simulink model "poleVaultSim"  (R2024a)
settings: Solver=VariableStepAuto  StartTime=0.0  StopTime=4  MaxStep=.0002  RelTol=1e-3  EnableMultiTasking=on
undefined symbols (not defined in the file or in its folder): k, theta0
libraries: simulink_extras x4
settings Model: PauseTimes=1.31  PacingRate=0.500000  Creator=amitraj  LastModifiedBy=grouleau
settings SolverCC: AlgebraicLoopSolver=TrustRegion
settings OptimizationCC: LifeSpan=inf
settings DebuggingCC: UnconnectedInputMsg=warning  UnconnectedOutputMsg=warning  UnconnectedLineMsg=warning  SFUnexpectedBacktrackingDiag=warning  SFNoUnconditionalDefaultTransitionDiag=warning  ArithmeticOperatorsInVariantConditions=warning
settings ModelReferenceCC: EnableRefExpFcnMdlSchedulingChecks=on
settings SFSimCC: SimUseLocalCustomCode=off  CustomCodeUndefinedFunction=UseInterfaceOnly
settings RTWCC: RTWUseLocalCustomCode=off  GPUComputeCapability=3.5
settings CodeAppCC: StateflowObjectComments=on
settings GRTTargetCC: TargetLangStandard=C89/C90 (ANSI)
settings ConfigComp: CovMetricSettings=dw  CovSaveCumulativeToWorkspaceVar=on  CovSaveSingleToWorkspaceVar=on  CovExternalEMLEnable=off

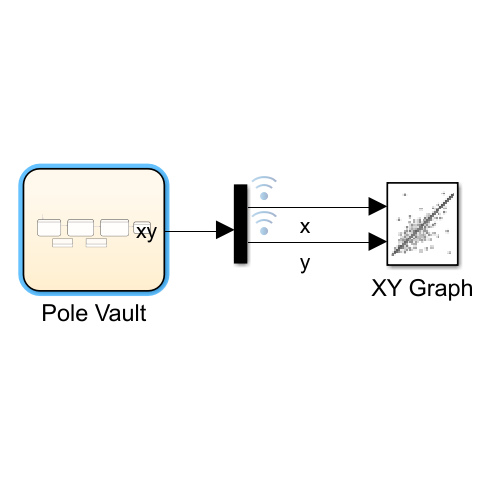
[thumbnail: Simulink's stored preview of the top-level diagram]
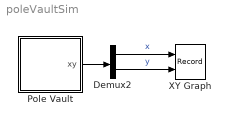
== system poleVaultSim ==
  Demux2 : Demux  Outputs=2
  Pole Vault : Stateflow chart  TreatAsAtomicUnit=on
  XY Graph : Record  FileSettingsInternal="{\"entries\":[{\"content\":{\"excelSettings\":{\"content\":{},\"type\":\"Streamout.ExcelSettings\"}},\"type\":\"Streamout.FileSettingStorage\",\"uuid\":\"\"}],\"packageUris\":[\"http:\\/\\/schema.mathworks.com\\/mf0\\/streamout_blocks\\/R2020a\"],\"version\":\"1.0\"}"  Layout=[1 1]  SignalsInternal="{\"entries\":[{\"content\":{\"signals\":[{\"content\":{\"blockPath\":[],\"dimensions\":[1],\"domain\":\"\",\"lineColor\":\"#a2142f\",\"plots\":[ 1 ],\"port\":1,\"sid\":[\"\"],\"signalID\":1,\"signalName\":\"x\"},\"type\":\"RecordBlkView.Signal\",\"uuid\":\"\"},{\"content\":{\"blockPath\":[],\"dimensions\":[1],\"domain\":\"\",\"lineColor\":\"#139fff\",\"plots\":[ 1 ],\"port\":2,\"sid\":[\"\"],\"signalID\":2,\"signalName\":\"y\"},\"type\":\"RecordBlkView.Signal\",\"uuid\":\"\"}]},\"type\":\"RecordBlkView.InputSignals\",\"uuid\":\"\"}],\"packageUris\":[\"http:\\/\\/schema.mathworks.com\\/mf0\\/streamout_blocks\\/R2020a\"],\"version\":\"1.0\"}"  VisualizationBindings="{\"xyplotplugin\":{\"info\":[{\"series\":[{\"bindingParametersList\":[{\"parameter\":\"X-Axis\",\"signalID\":1,\"signalName\":\"x\"},{\"parameter\":\"Y-Axis\",\"signalID\":2,\"signalName\":\"y\"}],\"seriesID\":0}],\"subplotID\":1}]}}"  CompatibilityTag=XY  st=-1
  wires:
  Demux2/1 -> XY Graph/1  "x"
  Demux2/2 -> XY Graph/2  "y"
  Pole Vault/1(xy) -> Demux2/1

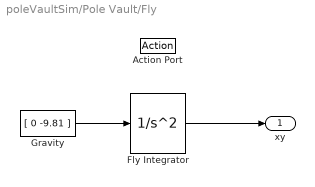
== system poleVaultSim/Pole Vault/Fly ==
  Action Port : ActionPort
      settings: CopyFcn=Stateflow.SLINSF.SimulinkMan.removeBlockPreDeleteFcn  PreDeleteFcn=Stateflow.SLINSF.SimulinkMan.unsafePredeleteFcn
  Fly Integrator : SecondOrderIntegrator  StateNameX='x'  StateNameDXDT='dx'  ShowOutput=x
  Gravity : Constant  Value=[ 0 -9.81 ]
  xy : Outport
  wires:
  Gravity/1 -> Fly Integrator/1
  Fly Integrator/1 -> xy/1

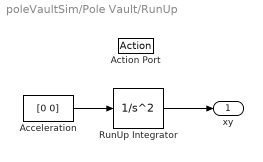
== system poleVaultSim/Pole Vault/RunUp ==
  Action Port : ActionPort
      settings: CopyFcn=Stateflow.SLINSF.SimulinkMan.removeBlockPreDeleteFcn  PreDeleteFcn=Stateflow.SLINSF.SimulinkMan.unsafePredeleteFcn
  Acceleration : Constant  Value=[0 0]
  RunUp Integrator : SecondOrderIntegrator  ICX=[10 1]  StateNameX='x'  ICDXDT=[-10 0]  StateNameDXDT='dx'  ShowOutput=x
      settings: AttributesFormatString=|
      | Initial Position: %<ICX>
      | Initial Velocity%<ICDXDT>
  xy : Outport
  wires:
  Acceleration/1 -> RunUp Integrator/1
  RunUp Integrator/1 -> xy/1

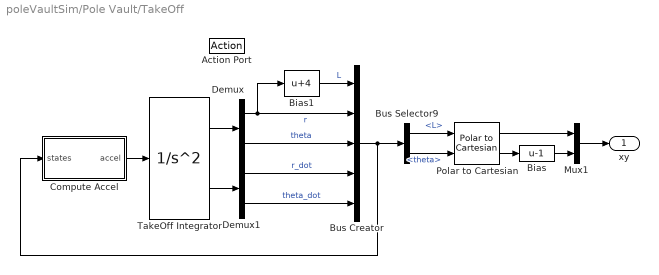
== system poleVaultSim/Pole Vault/TakeOff ==
  Action Port : ActionPort
      settings: CopyFcn=Stateflow.SLINSF.SimulinkMan.removeBlockPreDeleteFcn  PreDeleteFcn=Stateflow.SLINSF.SimulinkMan.unsafePredeleteFcn
  Bias : Bias  Bias=-1  SaturateOnIntegerOverflow=off
  Bias1 : Bias  Bias=4  SaturateOnIntegerOverflow=off
  Bus Creator : BusCreator  Inputs=5
  Bus Selector9 : BusSelector  OutputSignals=L,theta
  Compute Accel : Subsystem
  Demux : Demux  Outputs=2
  Demux1 : Demux  Outputs=2
  Mux1 : Mux  Inputs=2
  Polar to Cartesian : simulink_extras/Transformations/Polar to Cartesian
  TakeOff Integrator : SecondOrderIntegrator  StateNameX='x'  StateNameDXDT='dx'
  xy : Outport
  wires:
  Compute Accel/1(accel) -> TakeOff Integrator/1
  Bias/1 -> Mux1/2
  Demux1/1 -> Bus Creator/4  "r_dot"
  Polar to Cartesian/2 -> Bias/1
  Bus Selector9/1 -> Polar to Cartesian/1  "<L>"
  Mux1/1 -> xy/1
  Bus Selector9/2 -> Polar to Cartesian/2  "<theta>"
  TakeOff Integrator/1 -> Demux/1
  Polar to Cartesian/1 -> Mux1/1
  Bias1/1 -> Bus Creator/1  "L"
  Demux1/2 -> Bus Creator/5  "theta_dot"
  Bus Creator/1 -> Compute Accel/1(states), Bus Selector9/1
  Demux/1 -> Bus Creator/2, Bias1/1  "r"
  Demux/2 -> Bus Creator/3  "theta"
  TakeOff Integrator/2 -> Demux1/1

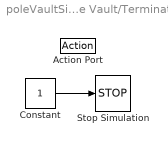
== system poleVaultSim/Pole Vault/Terminate ==
  Action Port : ActionPort
      settings: CopyFcn=Stateflow.SLINSF.SimulinkMan.removeBlockPreDeleteFcn  PreDeleteFcn=Stateflow.SLINSF.SimulinkMan.unsafePredeleteFcn
  Constant : Constant
  Stop Simulation : Stop
  wires:
  Constant/1 -> Stop Simulation/1

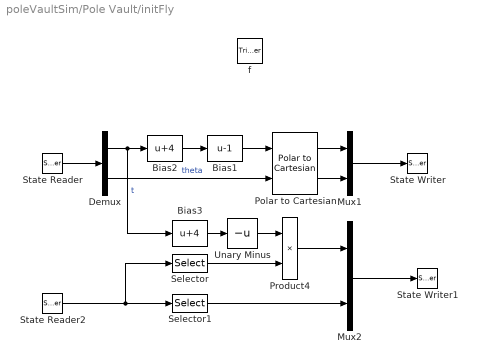
== system poleVaultSim/Pole Vault/initFly ==
  f : TriggerPort  TriggerType=function-call  VariantControl=(inherit)
      settings: CopyFcn=Stateflow.SLINSF.SimulinkMan.removeBlockPreDeleteFcn  PreDeleteFcn=Stateflow.SLINSF.SimulinkMan.unsafePredeleteFcn
  Bias1 : Bias  Bias=-1  SaturateOnIntegerOverflow=off
  Bias2 : Bias  Bias=4  SaturateOnIntegerOverflow=off
  Bias3 : Bias  Bias=4  SaturateOnIntegerOverflow=off
  Demux : Demux  Outputs=2
  Mux1 : Mux  Inputs=2
  Mux2 : Mux  Inputs=2
  Polar to Cartesian : simulink_extras/Transformations/Polar to Cartesian
  Product4 : Product
  Selector : Selector  InputPortWidth=2  IndexOptions=Index vector (dialog)  Indices=2  OutputSizes=1
  Selector1 : Selector  InputPortWidth=2  IndexOptions=Index vector (dialog)  Indices=1  OutputSizes=1
  State Reader : StateReader  StateOwnerBlock=../../TakeOff/TakeOff Integrator  StateName=x
  State Reader2 : StateReader  StateOwnerBlock=../../TakeOff/TakeOff Integrator  StateName=dx
  State Writer : StateWriter  StateOwnerBlock=../../Fly/Fly Integrator  StateName=x
  State Writer1 : StateWriter  StateOwnerBlock=../../Fly/Fly Integrator  StateName=dx
  Unary Minus : UnaryMinus
  wires:
  Bias2/1 -> Bias1/1
  Polar to Cartesian/1 -> Mux1/1
  Mux1/1 -> State Writer/1
  Bias1/1 -> Polar to Cartesian/1
  Polar to Cartesian/2 -> Mux1/2
  Demux/2 -> Polar to Cartesian/2  "theta"
  Product4/1 -> Mux2/1
  Selector1/1 -> Mux2/2
  Bias3/1 -> Unary Minus/1
  Mux2/1 -> State Writer1/1
  Unary Minus/1 -> Product4/1
  Demux/1 -> Bias3/1, Bias2/1  "t"
  State Reader/1 -> Demux/1
  Selector/1 -> Product4/2
  State Reader2/1 -> Selector/1, Selector1/1

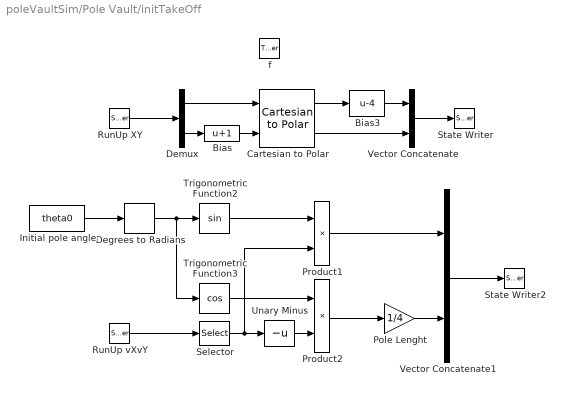
== system poleVaultSim/Pole Vault/initTakeOff ==
  f : TriggerPort  TriggerType=function-call  VariantControl=(inherit)
      settings: CopyFcn=Stateflow.SLINSF.SimulinkMan.removeBlockPreDeleteFcn  PreDeleteFcn=Stateflow.SLINSF.SimulinkMan.unsafePredeleteFcn
  Bias : Bias  Bias=1  SaturateOnIntegerOverflow=off
  Bias3 : Bias  Bias=-4  SaturateOnIntegerOverflow=off
  Cartesian to Polar : simulink_extras/Transformations/Cartesian to Polar
  Degrees to Radians : simulink_extras/Transformations/Degrees to Radians
  Demux : Demux  Outputs=2
  Initial pole angle : Constant  Value=theta0
  Pole Lenght : Gain  Gain=1/4
  Product1 : Product
  Product2 : Product
  RunUp XY : StateReader  StateOwnerBlock=../../RunUp/RunUp Integrator  StateName=x
  RunUp vXvY : StateReader  StateOwnerBlock=../../RunUp/RunUp Integrator  StateName=dx
  Selector : Selector  InputPortWidth=2  IndexOptions=Index vector (dialog)  Indices=1  OutputSizes=1
  State Writer : StateWriter  StateOwnerBlock=../../TakeOff/TakeOff Integrator  StateName=x
  State Writer2 : StateWriter  StateOwnerBlock=../../TakeOff/TakeOff Integrator  StateName=dx
  Trigonometric Function2 : Trigonometry
  Trigonometric Function3 : Trigonometry  Operator=cos
  Unary Minus : UnaryMinus
  Vector Concatenate : Concatenate
  Vector Concatenate1 : Concatenate
  wires:
  Unary Minus/1 -> Product2/2
  Product2/1 -> Pole Lenght/1
  RunUp vXvY/1 -> Selector/1
  Trigonometric Function3/1 -> Product2/1
  Trigonometric Function2/1 -> Product1/1
  Cartesian to Polar/1 -> Bias3/1
  Initial pole angle/1 -> Degrees to Radians/1
  Demux/1 -> Cartesian to Polar/1
  Demux/2 -> Bias/1
  Selector/1 -> Product1/2, Unary Minus/1
  Bias/1 -> Cartesian to Polar/2
  Pole Lenght/1 -> Vector Concatenate1/2
  RunUp XY/1 -> Demux/1
  Bias3/1 -> Vector Concatenate/1
  Cartesian to Polar/2 -> Vector Concatenate/2
  Vector Concatenate/1 -> State Writer/1
  Product1/1 -> Vector Concatenate1/1
  Vector Concatenate1/1 -> State Writer2/1
  Degrees to Radians/1 -> Trigonometric Function3/1, Trigonometric Function2/1

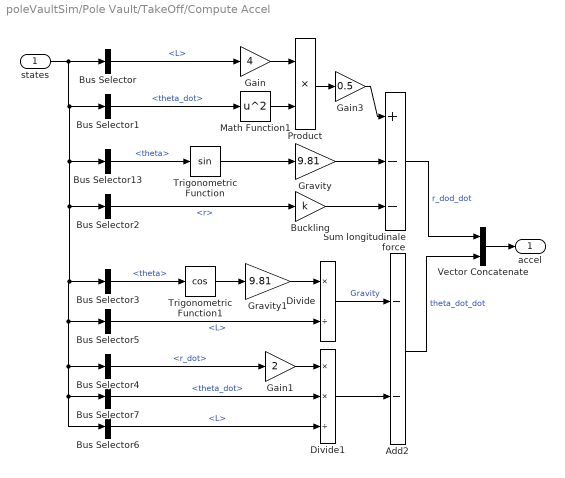
== system poleVaultSim/Pole Vault/TakeOff/Compute Accel ==
  states : Inport
  Add2 : Sum  Inputs=--
  Buckling : Gain  Gain=k
  Bus Selector : BusSelector  OutputSignals=L
  Bus Selector1 : BusSelector  OutputSignals=theta_dot
  Bus Selector13 : BusSelector  OutputSignals=theta
  Bus Selector2 : BusSelector  OutputSignals=r
  Bus Selector3 : BusSelector  OutputSignals=theta
  Bus Selector4 : BusSelector  OutputSignals=r_dot
  Bus Selector5 : BusSelector  OutputSignals=L
  Bus Selector6 : BusSelector  OutputSignals=L
  Bus Selector7 : BusSelector  OutputSignals=theta_dot
  Divide : Product  Inputs=*/
  Divide1 : Product  Inputs=**/
  Gain : Gain  Gain=4
  Gain1 : Gain  Gain=2
  Gain3 : Gain  Gain=0.5
  Gravity : Gain  Gain=9.81
  Gravity1 : Gain  Gain=9.81
  Math Function1 : Math  Operator=square  SignedPower=on
  Product : Product
  Sum longitudinale force : Sum  Inputs=+--
  Trigonometric Function : Trigonometry
  Trigonometric Function1 : Trigonometry  Operator=cos
  Vector Concatenate : Concatenate
  accel : Outport
  wires:
  Bus Selector2/1 -> Buckling/1  "<r>"
  Bus Selector/1 -> Gain/1  "<L>"
  Bus Selector1/1 -> Math Function1/1  "<theta_dot>"
  Gain3/1 -> Sum longitudinale force/1
  Gain/1 -> Product/1
  Gravity/1 -> Sum longitudinale force/2
  Buckling/1 -> Sum longitudinale force/3
  Trigonometric Function/1 -> Gravity/1
  Product/1 -> Gain3/1
  Math Function1/1 -> Product/2
  Sum longitudinale force/1 -> Vector Concatenate/1  "r_dod_dot"
  Bus Selector13/1 -> Trigonometric Function/1  "<theta>"
  Trigonometric Function1/1 -> Gravity1/1
  Gain1/1 -> Divide1/1
  Gravity1/1 -> Divide/1
  Divide1/1 -> Add2/2
  Divide/1 -> Add2/1  "Gravity"
  Bus Selector7/1 -> Divide1/2  "<theta_dot>"
  states/1 -> Bus Selector2/1, Bus Selector3/1, Bus Selector6/1, Bus Selector7/1, Bus Selector4/1, Bus Selector5/1, Bus Selector13/1, Bus Selector1/1, Bus Selector/1
  Bus Selector3/1 -> Trigonometric Function1/1  "<theta>"
  Bus Selector5/1 -> Divide/2  "<L>"
  Bus Selector4/1 -> Gain1/1  "<r_dot>"
  Bus Selector6/1 -> Divide1/3  "<L>"
  Add2/1 -> Vector Concatenate/2  "theta_dot_dot"
  Vector Concatenate/1 -> accel/1

== stateflow chart poleVaultSim/Pole Vault ==
  state RunUp
  state TakeOff
  state Fly
  state Terminate
  state initTakeOff [function]
  state initFly [function]
  (default) -> RunUp
  RunUp -> TakeOff : [RunUp.x(1) < 3.4641]
      | {initTakeOff;}
  Fly -> Terminate : [Fly.x(2)<=0]
  TakeOff -> Fly : [TakeOff.x(2)>pi/2]
      | {initFly;}
  data: sf_internal_action_state_placeholder_data local double size=1 =0; x local; sf_internal_action_state_placeholder_data local double size=1 =0; x local; sf_internal_action_state_placeholder_data local double size=1 =0; x local; sf_internal_action_state_placeholder_data local double size=1 =0; xy output
